simulink model "adaptiv6"  (Simulink 7.8)
settings: Solver=ode45  StartTime=0.0  StopTime=10.0  RelTol=1e-3
values from neighbouring files (symbols this model uses):
  n_koeff = 32    [adaptiv_4.m]    (also in adaptiv_5.m; adaptiv_6.m)
  Ts = 1/fs    (= 6.25e-05)    [G722_1.m]    (also in adaptiv_2.m = 0.001; adaptiv_3.m = 0.001; adaptiv_4.m = 0.001; adaptiv_5.m = 0.001)
  ts = (0:length(xs)-1)/250    [adaptiv_4.m]    (also in adaptiv_5.m; adaptiv_6.m)
  tsf = (0:length(xs)-1)/300    [adaptiv_5.m]    (also in adaptiv_6.m)
  xs = interp1(0:length(xs)-1, xs, 0:0.25:length(xs)-1,'spline')    [adaptiv_4.m]    (also in adaptiv_5.m; adaptiv_6.m)
  xsf = xs    [adaptiv_5.m]    (also in adaptiv_6.m)
libraries: simulink x2, dspadpt3 x1
settings Model: Creator=svenhoffmann  LastModifiedBy=josef  ExtModeAutoUpdateStatusClock=off
settings DataIOCC: SignalLoggingName=sigsOut
settings DebuggingCC: SaveWithParameterizedLinksMsg=none  SignalResolutionControl=TryResolveAllWithWarning  SolverPrmCheckMsg=none  MultiTaskDSMMsg=warning  MultiTaskCondExecSysMsg=none  StrictBusMsg=None
settings HardwareCC: TargetUnknown=on
settings RTWCC: IncludeERTFirstTime=on

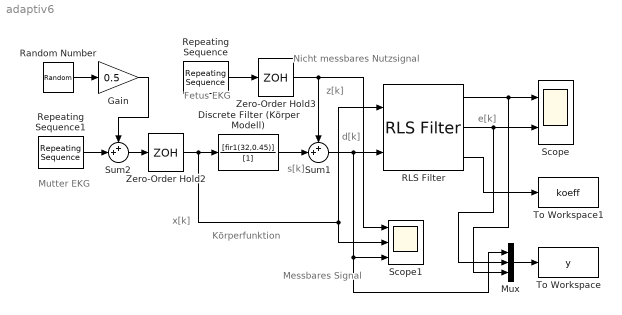
== system adaptiv6 ==
  note: Nicht messbares
      | Nutzsignal
  note: Messbares
      | Signal
  note: Körperfunktion
  note: Fetus EKG
  note: Mutter EKG
  note: d[k]
  note: s[k]
  note: z[k]
  note: x[k]
  note: e[k]
  Discrete Filter (Körper Modell) : DiscreteFilter  Numerator=[fir1(32,0.45)]  Denominator=[1]  SampleTime=Ts
  Gain : Gain  Gain=0.5  SaturateOnIntegerOverflow=on  OutDataTypeStr=Inherit: Same as input  ParamDataTypeStr=Inherit: Same as input
  Mux : Mux  Inputs=3
  RLS Filter : dspadpt3/RLS Filter  L=n_koeff  lambdaflag=Dialog  lambda=1.0  addnparflag=off  ic=0  delta=0.1  Adapt=off  resetflag=None  weights=on
  Random Number : RandomNumber  SampleTime=0
  Repeating Sequence : simulink/Sources/Repeating Sequence  rep_seq_t=[tsf]  rep_seq_y=[xsf]*0.5
  Repeating Sequence1 : simulink/Sources/Repeating Sequence  rep_seq_t=[ts]  rep_seq_y=[xs]
  Scope : Scope  NumInputPorts=2
      settings: YMin=-6~-0.6  YMax=7~0.7  SaveName=ScopeData2
  Scope1 : Scope  NumInputPorts=3
      settings: YMin=-5~-30~-5  YMax=7.5~30~5
  Sum1 : Sum  Inputs=++|  SaturateOnIntegerOverflow=on
  Sum2 : Sum  Inputs=++|  SaturateOnIntegerOverflow=on
  To Workspace : ToWorkspace  VariableName=y  SampleTime=-1  SaveFormat=Array
  To Workspace1 : ToWorkspace  VariableName=koeff  SampleTime=-1  SaveFormat=Array
      settings: MaxDataPoints=1
  Zero-Order Hold2 : ZeroOrderHold  SampleTime=Ts
  Zero-Order Hold3 : ZeroOrderHold  SampleTime=Ts
  wires:
  Repeating Sequence/1 -> Zero-Order Hold3/1
  Discrete Filter (Körper Modell)/1 -> Sum1/2
  Sum1/1 -> Mux/1, Scope1/3, RLS Filter/2
  RLS Filter/1 -> Scope/1, Mux/3
  RLS Filter/2 -> Scope/2, Mux/2
  RLS Filter/3 -> To Workspace1/1
  Mux/1 -> To Workspace/1
  Repeating Sequence1/1 -> Sum2/2
  Random Number/1 -> Gain/1
  Gain/1 -> Sum2/1
  Zero-Order Hold2/1 -> Scope1/2, RLS Filter/1, Discrete Filter (Körper Modell)/1
  Zero-Order Hold3/1 -> Sum1/1, Scope1/1
  Sum2/1 -> Zero-Order Hold2/1
